simulink model "Longitudinal_Simulink_MaskedParameter_WithOutput_02"  (Simulink 7.1)
settings: Solver=ode45  StartTime=0.0  StopTime=10.0  RelTol=1e-3
libraries: vrlib x2
settings Model: Creator=Meisel  LastModifiedBy=Meisel

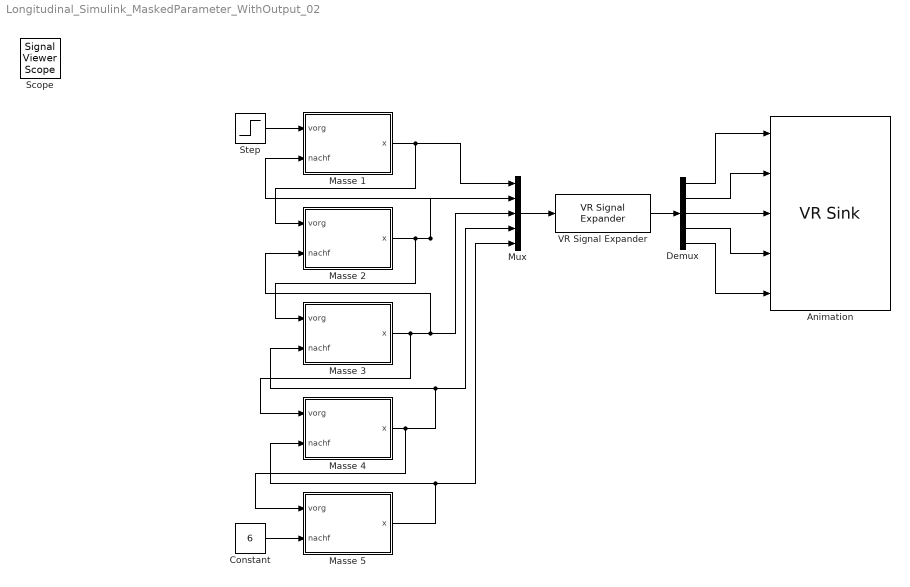
== system Longitudinal_Simulink_MaskedParameter_WithOutput_02 ==
  Animation : vrlib/VR Sink  SampleTime=0.01  ViewEnable=on  RemoteChange=off  RemoteView=on  FieldsWritten=m05.translation.3.1.double#m04.translation.3.1.double#m03.translation.3.1.double#m02.translation.3.1.double#m01.translation.3.1.double  WorldFileName=Massen_5.WRL  AutoView=off  VideoDimensions=[]  FigureProperties="{'Position', 'Name', 'Viewpoint', 'CameraBound', 'CameraDirection', 'CameraPosition', 'CameraUpVector', 'ZoomFactor', 'Antialiasing', 'Headlight', 'Lighting', 'NavPanel', 'StatusBar', 'ToolBar', 'Textures', 'Transparency', 'Wireframe', 'NavZones', 'NavMode', 'NavSpeed', 'Record2DCompressMethod', 'Record2DCompressQuality', 'Record2D', 'Record2DFileName', 'Record2DFPS'; [9.2000000000000000e+001  1.2400000000000000e+002  4.9100000000000000e+002  1.8200000000000000e+002], '', '_untitled_2', 'on', [5.2633573936155620e-001 -1.8738127758298598e-001 -8.2937262209581786e-001], [4.6106517249297135e-001  4.9665536299408264e-001 -9.6042888045995545e-001], [1.0040389152691827e-001  9.8228725778733783e-001 -1.5821125672619779e-001], [1.0000000000000000e+000], 'off', 'on', 'on', 'halfbar', 'off', 'on', 'on', 'on', 'off', 'off', 'examine', 'normal', 'auto', [7.5000000000000000e+001], 'off', '%f_anim_%n.avi', [1.5000000000000000e+001]}"
  Constant : Constant  Value=6  OutDataType=sfix(16)  OutScaling=2^0
  Demux : Demux  Outputs=5
  Masse 1 : Subsystem  mask{Init_Pos=1}
      mask prompts: Init_Pos "Startposition"
  Masse 2 : Subsystem  mask{Init_Pos=2}
      mask prompts: Init_Pos "Startposition"
  Masse 3 : Subsystem  mask{Init_Pos=3}
      mask prompts: Init_Pos "Startposition"
  Masse 4 : Subsystem  mask{Init_Pos=4}
      mask prompts: Init_Pos "Startposition"
  Masse 5 : Subsystem  mask{Init_Pos=5}
      mask prompts: Init_Pos "Startposition"
  Mux : Mux  Inputs=5
  Step : Step  Time=0  After=0.5  SampleTime=0
  VR Signal Expander : vrlib/VR Signal Expander  SystemSampleTime=-1  outwidth=15  outidx=[13 10 7 4 1]
  Scope : SignalViewerScope  IOType=viewer  RefreshTime=0.035000
      settings: YMin=0  YMax=0.1
  wires:
  Masse 1/1(x) -> Mux/1, Masse 2/1(vorg)
  Step/1 -> Masse 1/1(vorg)
  Masse 2/1(x) -> Masse 3/1(vorg), Masse 1/2(nachf), Mux/2
  Masse 3/1(x) -> Masse 4/1(vorg), Masse 2/2(nachf), Mux/3
  Masse 4/1(x) -> Masse 5/1(vorg), Masse 3/2(nachf), Mux/4
  Masse 5/1(x) -> Masse 4/2(nachf), Mux/5
  Constant/1 -> Masse 5/2(nachf)
  Mux/1 -> VR Signal Expander/1
  VR Signal Expander/1 -> Demux/1
  Demux/1 -> Animation/1
  Demux/2 -> Animation/2
  Demux/3 -> Animation/3
  Demux/4 -> Animation/4
  Demux/5 -> Animation/5

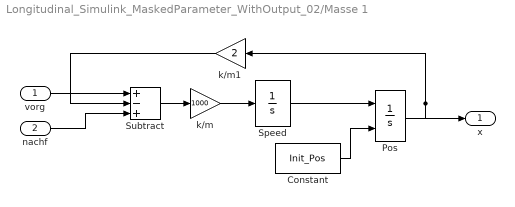
== system Longitudinal_Simulink_MaskedParameter_WithOutput_02/Masse 1 ==
  vorg : Inport  OutDataType=sfix(16)  OutScaling=2^0
  nachf : Inport  Port=2  OutDataType=sfix(16)  OutScaling=2^0
  Constant : Constant  Value=Init_Pos  OutDataType=sfix(16)  OutScaling=2^0
  Pos : Integrator  InitialConditionSource=external  InitialCondition=1
  Speed : Integrator
  Subtract : Sum  Inputs=+-+  OutDataType=sfix(16)  OutScaling=2^-10
  k/m : Gain  Gain=1000  ParameterDataType=sfix(16)  ParameterScaling=2^0  OutDataType=sfix(16)  OutScaling=2^0
  k/m1 : Gain  Orientation=left  Gain=2  ParameterDataType=sfix(16)  ParameterScaling=2^0  OutDataType=sfix(16)  OutScaling=2^0
  x : Outport  OutDataType=sfix(16)  OutScaling=2^0
  wires:
  Speed/1 -> Pos/1
  Subtract/1 -> k/m/1
  k/m/1 -> Speed/1
  Pos/1 -> x/1, k/m1/1
  nachf/1 -> Subtract/3
  vorg/1 -> Subtract/1
  k/m1/1 -> Subtract/2
  Constant/1 -> Pos/2

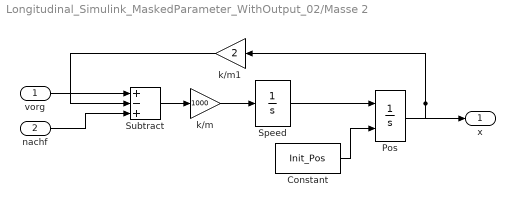
== system Longitudinal_Simulink_MaskedParameter_WithOutput_02/Masse 2 ==
  vorg : Inport  OutDataType=sfix(16)  OutScaling=2^0
  nachf : Inport  Port=2  OutDataType=sfix(16)  OutScaling=2^0
  Constant : Constant  Value=Init_Pos  OutDataType=sfix(16)  OutScaling=2^0
  Pos : Integrator  InitialConditionSource=external  InitialCondition=1
  Speed : Integrator
  Subtract : Sum  Inputs=+-+  OutDataType=sfix(16)  OutScaling=2^-10
  k/m : Gain  Gain=1000  ParameterDataType=sfix(16)  ParameterScaling=2^0  OutDataType=sfix(16)  OutScaling=2^0
  k/m1 : Gain  Orientation=left  Gain=2  ParameterDataType=sfix(16)  ParameterScaling=2^0  OutDataType=sfix(16)  OutScaling=2^0
  x : Outport  OutDataType=sfix(16)  OutScaling=2^0
  wires:
  Speed/1 -> Pos/1
  Subtract/1 -> k/m/1
  k/m/1 -> Speed/1
  Pos/1 -> x/1, k/m1/1
  nachf/1 -> Subtract/3
  vorg/1 -> Subtract/1
  k/m1/1 -> Subtract/2
  Constant/1 -> Pos/2

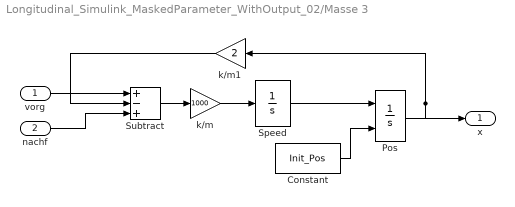
== system Longitudinal_Simulink_MaskedParameter_WithOutput_02/Masse 3 ==
  vorg : Inport  OutDataType=sfix(16)  OutScaling=2^0
  nachf : Inport  Port=2  OutDataType=sfix(16)  OutScaling=2^0
  Constant : Constant  Value=Init_Pos  OutDataType=sfix(16)  OutScaling=2^0
  Pos : Integrator  InitialConditionSource=external  InitialCondition=1
  Speed : Integrator
  Subtract : Sum  Inputs=+-+  OutDataType=sfix(16)  OutScaling=2^-10
  k/m : Gain  Gain=1000  ParameterDataType=sfix(16)  ParameterScaling=2^0  OutDataType=sfix(16)  OutScaling=2^0
  k/m1 : Gain  Orientation=left  Gain=2  ParameterDataType=sfix(16)  ParameterScaling=2^0  OutDataType=sfix(16)  OutScaling=2^0
  x : Outport  OutDataType=sfix(16)  OutScaling=2^0
  wires:
  Speed/1 -> Pos/1
  Subtract/1 -> k/m/1
  k/m/1 -> Speed/1
  Pos/1 -> x/1, k/m1/1
  nachf/1 -> Subtract/3
  vorg/1 -> Subtract/1
  k/m1/1 -> Subtract/2
  Constant/1 -> Pos/2

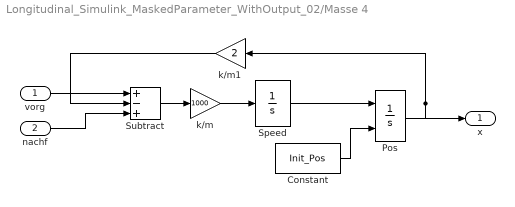
== system Longitudinal_Simulink_MaskedParameter_WithOutput_02/Masse 4 ==
  vorg : Inport  OutDataType=sfix(16)  OutScaling=2^0
  nachf : Inport  Port=2  OutDataType=sfix(16)  OutScaling=2^0
  Constant : Constant  Value=Init_Pos  OutDataType=sfix(16)  OutScaling=2^0
  Pos : Integrator  InitialConditionSource=external  InitialCondition=1
  Speed : Integrator
  Subtract : Sum  Inputs=+-+  OutDataType=sfix(16)  OutScaling=2^-10
  k/m : Gain  Gain=1000  ParameterDataType=sfix(16)  ParameterScaling=2^0  OutDataType=sfix(16)  OutScaling=2^0
  k/m1 : Gain  Orientation=left  Gain=2  ParameterDataType=sfix(16)  ParameterScaling=2^0  OutDataType=sfix(16)  OutScaling=2^0
  x : Outport  OutDataType=sfix(16)  OutScaling=2^0
  wires:
  Speed/1 -> Pos/1
  Subtract/1 -> k/m/1
  k/m/1 -> Speed/1
  Pos/1 -> x/1, k/m1/1
  nachf/1 -> Subtract/3
  vorg/1 -> Subtract/1
  k/m1/1 -> Subtract/2
  Constant/1 -> Pos/2

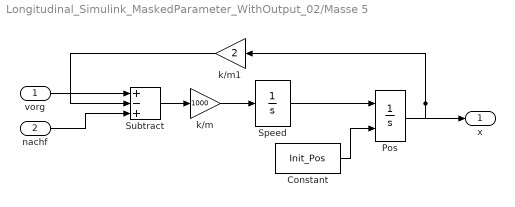
== system Longitudinal_Simulink_MaskedParameter_WithOutput_02/Masse 5 ==
  vorg : Inport  OutDataType=sfix(16)  OutScaling=2^0
  nachf : Inport  Port=2  OutDataType=sfix(16)  OutScaling=2^0
  Constant : Constant  Value=Init_Pos  OutDataType=sfix(16)  OutScaling=2^0
  Pos : Integrator  InitialConditionSource=external  InitialCondition=1
  Speed : Integrator
  Subtract : Sum  Inputs=+-+  OutDataType=sfix(16)  OutScaling=2^-10
  k/m : Gain  Gain=1000  ParameterDataType=sfix(16)  ParameterScaling=2^0  OutDataType=sfix(16)  OutScaling=2^0
  k/m1 : Gain  Orientation=left  Gain=2  ParameterDataType=sfix(16)  ParameterScaling=2^0  OutDataType=sfix(16)  OutScaling=2^0
  x : Outport  OutDataType=sfix(16)  OutScaling=2^0
  wires:
  Speed/1 -> Pos/1
  Subtract/1 -> k/m/1
  k/m/1 -> Speed/1
  Pos/1 -> x/1, k/m1/1
  nachf/1 -> Subtract/3
  vorg/1 -> Subtract/1
  k/m1/1 -> Subtract/2
  Constant/1 -> Pos/2
